simulink model "test_evaporator"  (R2021b)
settings: Solver=VariableStepAuto  StartTime=0.0  StopTime=40000  RelTol=1e-3
settings Model: Creator=Edwar  LastModifiedBy=Edwar

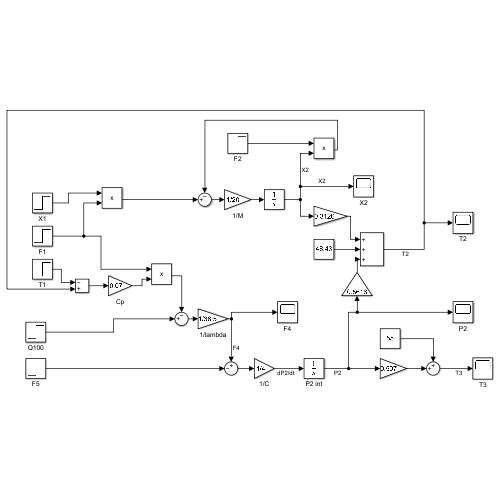
[thumbnail: Simulink's stored preview of the top-level diagram]
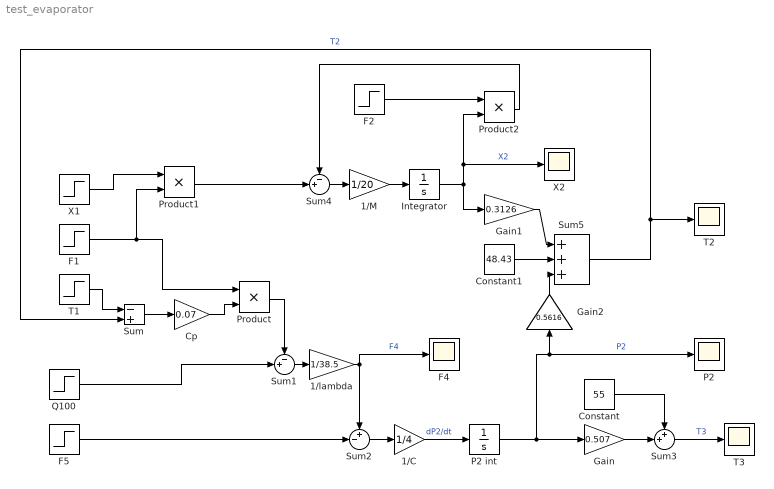
== system test_evaporator ==
  1/C : Gain  Gain=1/4
  1/M : Gain  Gain=1/20
  1/lambda : Gain  Gain=1/38.5
  Constant : Constant  Value=55
  Constant1 : Constant  Value=48.43
  Cp : Gain  Gain=0.07
  F1 : Step  SampleTime=0
  F2 : Step  SampleTime=0
  F4 : Scope
  F5 : Step  SampleTime=0
  Gain : Gain  Gain=0.507
  Gain1 : Gain  Gain=0.3126
  Gain2 : Gain  Gain=0.5616
  Integrator : Integrator
  P2 : Scope
  P2 int : Integrator
  Product : Product
  Product1 : Product
  Product2 : Product
  Q100 : Step  SampleTime=0
  Sum : Sum  Inputs=-+
  Sum1 : Sum  Inputs=-+|
  Sum2 : Sum  Inputs=+-|
  Sum3 : Sum  Inputs=++|
  Sum4 : Sum  Inputs=-+|
  Sum5 : Sum  Inputs=+++
  T1 : Step  SampleTime=0
  T2 : Scope
  T3 : Scope
  X1 : Step  SampleTime=0
  X2 : Scope
  wires:
  T1/1 -> Sum/1
  Sum/1 -> Cp/1
  Cp/1 -> Product/2
  F1/1 -> Product1/2, Product/1
  Q100/1 -> Sum1/2
  Product/1 -> Sum1/1
  F5/1 -> Sum2/2
  Sum2/1 -> 1/C/1
  1/C/1 -> P2 int/1  "dP2/dt"
  P2 int/1 -> Gain2/1, P2/1, Gain/1  "P2"
  Gain/1 -> Sum3/2
  Constant/1 -> Sum3/1
  Sum3/1 -> T3/1  "T3"
  Sum1/1 -> 1/lambda/1
  1/lambda/1 -> F4/1, Sum2/1  "F4"
  X1/1 -> Product1/1
  Integrator/1 -> X2/1, Product2/2, Gain1/1  "X2"
  F2/1 -> Product2/1
  Product1/1 -> Sum4/2
  Product2/1 -> Sum4/1
  Sum4/1 -> 1/M/1
  1/M/1 -> Integrator/1
  Constant1/1 -> Sum5/2
  Sum5/1 -> T2/1, Sum/2  "T2"
  Gain1/1 -> Sum5/1
  Gain2/1 -> Sum5/3
